simulink model "CAMFC2_04_Quad_03_R2017a"  (R2017a)
settings: Solver=ode45  StartTime=0.0  StopTime=360  RelTol=1e-3  EnableMultiTasking=on
InitFcn:
  | constant_CAMFC2_04_Quad_03
values from neighbouring files (symbols this model uses):
  alpha = 0.1    [constant_CAMFC2_01_WMR01.m]    (also in constant_CAMFC2_04_Comp.m = 0.01; constant_CAMFC2_04_Quad_03.m; constant_CAMFC2_04_Simple.m = 0.01; constant_CAMFC2_04_Simple_DoubleIntegrator.m = 0.01)
  AN = [     0 1 0 0 ... (first row only)    [constant_CAMFC2_01_WMR01.m]    (also in constant_CAMFC2_04_Comp.m = [     0 1 0 0 1; constant_CAMFC2_04_Quad_03.m; constant_CAMFC2_04_Simple.m; constant_CAMFC2_04_Simple_DoubleIntegrator.m)
  B = eye(n)    [constant_CAMFC2_01_WMR01.m]    (also in constant_CAMFC2_04_Quad_03.m; constant_CAMFC2_Quad_New_02.m)
  BBT_inv = ((B'*B)^(-1))*B'    [constant_CAMFC2_04_Quad_03.m]    (also in constant_CAMFC2_Quad_New_02.m)
  Beta = 0.2    [constant_CAMFC2_04_Quad_03.m]    (also in constant_CAMFC2_Quad_New_02.m = 0.1)
  BN = [     1 0 0 0 ... (first row only)    [constant_CAMFC2_01_WMR01.m]    (also in constant_CAMFC2_04_Comp.m = [     0 0 0 0 0; constant_CAMFC2_04_Quad_03.m; constant_CAMFC2_04_Simple.m; constant_CAMFC2_04_Simple_DoubleIntegrator.m)
  Bv = eye(n0)    [constant_CAMFC2_04_Quad_03.m]
  BvBT_inv = ((Bv'*Bv)^(-1))*Bv'    [constant_CAMFC2_04_Quad_03.m]
  chi = [0 0 0 0 ... (first row only)    [constant_CAMFC2_01_WMR01.m]    (also in constant_CAMFC2_04_Comp.m = X_m*ones(n0,1); constant_CAMFC2_04_Quad_03.m = X_m*ones(n0,1); constant_CAMFC2_04_Simple.m = X_m*ones(n0,1); constant_CAMFC2_04_Simple_DoubleIntegrator.m = X_m*ones(n0,1))
  epsilon_struct = struct('data',epsilon_InitVal)    [constant_CAMFC2_01_WMR01.m]    (also in constant_CAMFC2_04_Comp.m; constant_CAMFC2_04_Quad_03.m; constant_CAMFC2_04_Simple.m; constant_CAMFC2_04_Simple_DoubleIntegrator.m)
  gama1 = 1e4*diag([1e-6*ones(2,1);1e0*ones(2,1)])    [constant_CAMFC2_01_WMR01.m]    (also in constant_CAMFC2_04_Comp.m = 1e+3*diag([1e-6;1e-0]); constant_CAMFC2_04_Quad_03.m = 1e+2*diag(1e-0*ones(n0,1)); constant_CAMFC2_04_Simple.m = 1e+2*diag([1e-0;1e-0]); constant_CAMFC2_04_Simple_Formation.m = 1e+2*diag([1e-0;1e-0]))
  gama2 = 1e-2*diag([1e-6*ones(2,1);1e0*ones(2,1)])    [constant_CAMFC2_01_WMR01.m]    (also in constant_CAMFC2_04_Comp.m = 1e+0*diag([1e-6;1e-0]); constant_CAMFC2_04_Quad_03.m = 1e+0*diag(1e-0*ones(n0,1)); constant_CAMFC2_04_Simple.m = 1e+1*diag([1e-0;1e-0]); constant_CAMFC2_04_Simple_Formation.m = 1e+1*diag([1e-0;1e-0]))
  gamma_0 = 1e+0*diag([1e-0*ones(n0,1);1e-0*ones(n0,1)])    [constant_CAMFC2_04_Quad_03.m]    (also in constant_CAMFC2_Quad_New_02.m = 1e-2*diag([1e-6*ones(n0,1);1e-0*ones(n0,1)]))
  gamma_0v = 1e-0*diag(1e-0*ones(n0,1))    [constant_CAMFC2_04_Quad_03.m]
  gamma_1 = 1e+2*diag([1e-0*ones(n0,1);1e-0*ones(n0,1)])    [constant_CAMFC2_04_Quad_03.m]    (also in constant_CAMFC2_Quad_New_02.m = 1e+1*diag([1e-6*ones(n0,1);1e-0*ones(n0,1)]))
  gamma_1v = 1e+2*diag(1e-0*ones(n0,1))    [constant_CAMFC2_04_Quad_03.m]
  ge = 9.81    [constant_CAMFC2_04_Comp.m]    (also in constant_CAMFC2_04_Quad_03.m; constant_CAMFC2_04_Simple.m; constant_CAMFC2_04_Simple_DoubleIntegrator.m; constant_CAMFC2_04_Simple_DoubleIntegrator_02.m)
  H = L + BN    [constant_CAMFC2_01_WMR01.m]    (also in constant_CAMFC2_04_Comp.m; constant_CAMFC2_04_Quad_03.m; constant_CAMFC2_04_Simple.m; constant_CAMFC2_04_Simple_DoubleIntegrator.m)
  Init_Pos_Dif = 0.0    (= 0)    [constant_CAMFC2_04_Quad_03.m]
  J = 0.01    [constant_CAMFC2_01_WMR01.m]    (also in constant_CAMFC2_04_Quad_03.m = 1.0e-3 * diag([1 1 2],0); constant_CAMFC2_Quad_New_02.m = 1.2416e-3 * diag([1 1 2],0))
  k1 = 1    [constant_CAMFC2_01_WMR01.m]    (also in constant_CAMFC2_04_Comp.m; constant_CAMFC2_04_Quad_03.m = 50; constant_CAMFC2_04_Simple.m; constant_CAMFC2_04_Simple_DoubleIntegrator.m)
  k2 = 1    [constant_CAMFC2_01_WMR01.m]    (also in constant_CAMFC2_04_Comp.m; constant_CAMFC2_04_Quad_03.m; constant_CAMFC2_04_Simple.m; constant_CAMFC2_04_Simple_DoubleIntegrator.m)
  Ka = 0.1    [constant_CAMFC2_04_Quad_03.m]    (also in constant_CAMFC2_Quad_New_02.m = 0.01)
  Kd = 0.1    [constant_CAMFC2_04_Quad_03.m]    (also in constant_CAMFC2_Quad_New_02.m = 0.01)
  m = 6    [constant_CAMFC2_04_Quad_03.m]    (also in constant_CAMFC2_Quad_New_02.m)
  M = 1    [constant_CAMFC2_01_WMR01.m]    (also in constant_CAMFC2_04_Quad_03.m = 2; constant_CAMFC2_Quad_New_02.m = 2)
  N = 4    [constant_CAMFC2_01_WMR01.m]    (also in constant_CAMFC2_04_Comp.m = 5; constant_CAMFC2_04_Quad_03.m; constant_CAMFC2_04_Simple.m; constant_CAMFC2_04_Simple_DoubleIntegrator.m)
  n = 4    [constant_CAMFC2_01_WMR01.m]    (also in constant_CAMFC2_04_Comp.m = 2; constant_CAMFC2_04_Quad_03.m = 6; constant_CAMFC2_04_Simple.m = 2; constant_CAMFC2_04_Simple_DoubleIntegrator.m = 2)
  n0 = 2    [constant_CAMFC2_01_WMR01.m]    (also in constant_CAMFC2_04_Comp.m = 1; constant_CAMFC2_04_Quad_03.m = 3; constant_CAMFC2_04_Simple.m; constant_CAMFC2_04_Simple_DoubleIntegrator.m = 1)
  noise_amp = 0.1    [constant_CAMFC2_04_Quad_03.m]
  noise_frq = 1    [constant_CAMFC2_04_Quad_03.m]
  Observer_Gain = 100    [constant_CAMFC2_01_WMR01.m]    (also in constant_CAMFC2_04_Comp.m = 10; constant_CAMFC2_04_Quad_03.m = 1; constant_CAMFC2_04_Simple.m; constant_CAMFC2_04_Simple_DoubleIntegrator.m)
  Observer_Gain1 = 100    [constant_CAMFC2_01_WMR01.m]    (also in constant_CAMFC2_04_Comp.m = 10; constant_CAMFC2_04_Quad_03.m = 1; constant_CAMFC2_04_Simple.m; constant_CAMFC2_04_Simple_DoubleIntegrator.m)
  P_struct = struct('data',P_InitVal)    [constant_CAMFC2_01_WMR01.m]    (also in constant_CAMFC2_04_Comp.m; constant_CAMFC2_04_Quad_03.m; constant_CAMFC2_04_Simple.m; constant_CAMFC2_04_Simple_DoubleIntegrator.m)
  Q = 1e-0*eye(n)    [constant_CAMFC2_01_WMR01.m]    (also in constant_CAMFC2_04_Comp.m = 1.0e+2*eye(n); constant_CAMFC2_04_Quad_03.m = 1e-0*eye(n0); constant_CAMFC2_04_Simple.m = 1.0e+1*eye(n); constant_CAMFC2_04_Simple_Formation.m = 1.0e+1*eye(n))
  QR = 1e-0*eye(n)    [constant_CAMFC2_04_Quad_03.m]    (also in constant_CAMFC2_Quad_New_02.m = 1e+0*eye(n))
  Qv = 1e-0*eye(n0)    [constant_CAMFC2_04_Quad_03.m]
  R = 1e-0*eye(n)    [constant_CAMFC2_01_WMR01.m]    (also in constant_CAMFC2_04_Quad_03.m; constant_CAMFC2_Quad_New_02.m = 1e+0*eye(n))
  r_formX = 1.0    (= 1)    [constant_CAMFC2_04_Quad_03.m]    (also in constant_CAMFC2_Quad_New_02.m)
  r_formY = 1.0    (= 1)    [constant_CAMFC2_04_Quad_03.m]    (also in constant_CAMFC2_Quad_New_02.m)
  r_formZ = 0.5    [constant_CAMFC2_04_Quad_03.m]    (also in constant_CAMFC2_Quad_New_02.m = 1)
  rho1 = 1e-1    (= 0.1)    [constant_CAMFC2_01_WMR01.m]    (also in constant_CAMFC2_04_Comp.m = 1; constant_CAMFC2_04_Quad_03.m = 1; constant_CAMFC2_04_Simple.m = 1; constant_CAMFC2_04_Simple_DoubleIntegrator.m = 1)
  rho2 = 1e-3    (= 0.001)    [constant_CAMFC2_01_WMR01.m]    (also in constant_CAMFC2_04_Comp.m = 1; constant_CAMFC2_04_Quad_03.m = 1; constant_CAMFC2_04_Simple.m = 1; constant_CAMFC2_04_Simple_DoubleIntegrator.m = 10)
  rho_0 = 1e-0    (= 1)    [constant_CAMFC2_04_Quad_03.m]    (also in constant_CAMFC2_Quad_New_02.m = 0.01)
  rho_0v = 1e-0    (= 1)    [constant_CAMFC2_04_Quad_03.m]
  rho_1 = 1e-0    (= 1)    [constant_CAMFC2_04_Quad_03.m]    (also in constant_CAMFC2_Quad_New_02.m = 0.01)
  rho_1v = 1e-0    (= 1)    [constant_CAMFC2_04_Quad_03.m]
  Rv = 1e-0*eye(n0)    [constant_CAMFC2_04_Quad_03.m]
  T_struct = struct('data',T_InitVal)    [constant_CAMFC2_01_WMR01.m]    (also in constant_CAMFC2_04_Comp.m; constant_CAMFC2_04_Quad_03.m; constant_CAMFC2_04_Simple.m; constant_CAMFC2_04_Simple_DoubleIntegrator.m)
  Upsilon_M = Upsilon_m*ones(n,1)    [constant_CAMFC2_01_WMR01.m]    (also in constant_CAMFC2_04_Comp.m; constant_CAMFC2_04_Quad_03.m = Upsilon_m*ones(n0,1); constant_CAMFC2_04_Simple.m; constant_CAMFC2_04_Simple_DoubleIntegrator.m)
(part 3 of 4)

== matlab function CAMFC2_04_Quad_03_R2017a/Agent #2/Decenteralized Cooperaive Controller #2/Cooperative Position Controller #2/Module to compute Consensus Error #2 ==
  data: T_i input; x input; x0 input; ep output; AN parameter; BN parameter; N parameter; n0 parameter; Agent_Num input
function ep = fcn(T_i,x,x0,AN,BN,N,n0,Agent_Num)

Diff_Star_to0 = (T_i((Agent_Num+1),:))';
Diff_Star_to_Other = (eye(n0) * Diff_Star_to0 * ones(1,N))' - T_i(2:N+1,:);
Diff_Star_to_Other = Diff_Star_to_Other';

xp = zeros(n0,N);
for i=1:N
    xp(1:n0,i) = x((i-1)*n0+1:(i*n0));
end

%%
xp_own = zeros(n0,1);
xp_own(1:n0,1) = xp(1:n0,Agent_Num);

xp0 = x0;

xp_other = zeros(n0,N);
ep = zeros(n0,1);
ep(:,1) = ep(:,1) + ( BN(Agent_Num,Agent_Num)*(-(xp_own-xp0)+Diff_Star_to0) );

for i=1:N        
    xp_other(:,i) = xp(:,i);
    ep(:,1) = ep(:,1) + AN(Agent_Num,i)*(-(xp_own-xp_other(:,i))+Diff_Star_to_Other(:,i));
end

end

== matlab function CAMFC2_04_Quad_03_R2017a/Agent #2/Decenteralized Cooperaive Controller #2/Cooperative Position Controller #2/Observer T#2 ==
  data: T_struct parameter; T input; DT_i output; epsilon input; epsilon_struct parameter; H parameter; BN parameter; AN parameter; T_i input; Omega input; Upsilon_M parameter; epsilon_i output; N parameter; n0 parameter; Agent_Num input; Observer_Gain1 parameter; alpha parameter
function [DT_i,epsilon_i] = fcn(T_struct,T,epsilon,epsilon_struct,H,BN,AN,T_i,Omega, Upsilon_M,N,n0,Agent_Num,Observer_Gain1,alpha)

T_struct(1).data = T.t1;
T_struct(2).data = T.t2;
T_struct(3).data = T.t3;
T_struct(4).data = T.t4;

epsilon_struct(1).data = epsilon.eps1;
epsilon_struct(2).data = epsilon.eps2;
epsilon_struct(3).data = epsilon.eps3;
epsilon_struct(4).data = epsilon.eps4;

epsilon_i = + BN(Agent_Num,Agent_Num)*(T_i - Omega);
Sum2 = zeros(N+1,n0);
for i=1:N
    epsilon_i = epsilon_i + ( AN(Agent_Num,i) * (T_i - T_struct(i).data) );  
    Sum2 = Sum2 + ( H(i,Agent_Num) * epsilon_struct(i).data );
end

Sum21 = abs(Sum2) + alpha;
SGN2 = Sum2./Sum21;

DT_i = -Observer_Gain1*epsilon_i - SGN2*diag(Upsilon_M);

end

== matlab function CAMFC2_04_Quad_03_R2017a/Agent #2/Decenteralized Cooperaive Controller #2/Cooperative Position Controller #2/Observer x0_hat#2 ==
  data: x0_hat input; Dx0_hat_i output; x0_tilde input; H parameter; BN parameter; AN parameter; x0_hat_i input; x0 input; chi parameter; x0_tilde_i output; N parameter; Agent_Num input; Observer_Gain parameter; n0 parameter; alpha parameter
function [Dx0_hat_i,x0_tilde_i] = fcn(x0_hat,x0_tilde,H,BN,AN,x0_hat_i,x0,chi,N,Agent_Num,Observer_Gain,n0,alpha)

x0_tilde_i = + BN(Agent_Num,Agent_Num)*(x0_hat_i - x0);

if n0 == 1
    Sum2 = 0;
    for i=1:N
        x0_tilde_i = x0_tilde_i + ( AN(Agent_Num,i) * (x0_hat_i - x0_hat(i)) );  
        Sum2 = Sum2 + ( H(i,Agent_Num) * x0_tilde(i) );
    end    
else
    Sum2 = zeros(n0,1);
    for i=1:N
        x0_tilde_i = x0_tilde_i + ( AN(Agent_Num,i) * (x0_hat_i - x0_hat(((i-1)*n0+1):n0*i)) );  
        Sum2 = Sum2 + ( H(i,Agent_Num) * x0_tilde(((i-1)*n0+1):n0*i) );
    end
end

Sum21 = abs(Sum2) + alpha;
SGN2 = Sum2./Sum21;

Dx0_hat_i = -Observer_Gain*x0_tilde_i - diag(SGN2)*chi;

end

== matlab function CAMFC2_04_Quad_03_R2017a/Agent #2/Decenteralized Cooperaive Controller #2/Rotational AMFC #2/CARE ==
  data: P input; a_hat input; B parameter; R parameter; DP output; QR parameter
function DP = fcn(P,a_hat,B,R,QR)

DP = a_hat*P + P*a_hat' - P*B*R*B'*P + 2*QR;

end

== matlab function CAMFC2_04_Quad_03_R2017a/Agent #2/Decenteralized Cooperaive Controller #2/Rotational AMFC #2/Differentiator/Sliding differentiator ==
  data: u output; u1 input; e input; k1 parameter; alpha parameter
function u = fcn(u1,e,k1,alpha)

b=k1;

ABS = abs(e);
SGN = e ./ (ABS + alpha);
u = u1 - b*((ABS.^0.5).*SGN); 

end

== matlab function CAMFC2_04_Quad_03_R2017a/Agent #2/Decenteralized Cooperaive Controller #2/Rotational AMFC #2/Differentiator/Sliding differentiator1 ==
  data: Du1 output; e input; k2 parameter; alpha parameter
function Du1 = fcn(e,k2,alpha)

a=k2;

ABS = abs(e);
SGN = e ./ (ABS + alpha);
Du1 = - a*SGN;

end

== matlab function CAMFC2_04_Quad_03_R2017a/Agent #2/Decenteralized Cooperaive Controller #2/Rotational AMFC #2/g-Estimator ==
  data: sigma input; g_hat input; P input; rho_1 parameter; gamma_1 parameter; Dg_hat output
function Dg_hat = fcn(sigma,g_hat,P,rho_1,gamma_1)

Dg_hat = - gamma_1 * P * sigma - rho_1 * gamma_1 * g_hat;

end

== matlab function CAMFC2_04_Quad_03_R2017a/Agent #2/Decenteralized Cooperaive Controller #2/Rotational AMFC #2/A-Estimator ==
  data: sigma input; x input; P input; rho_0 parameter; gamma_0 parameter; Da_hat output; a_hat input
function Da_hat = fcn(sigma,x,P,rho_0,gamma_0,a_hat)

DVa_hat = - gamma_0 * P * diag(sigma) * (x - sigma) - rho_0 * gamma_0 * diag(a_hat);

Da_hat = diag(DVa_hat);

end

== matlab function CAMFC2_04_Quad_03_R2017a/Agent #2/Decenteralized Cooperaive Controller #2/Rotational AMFC #2/main ==
  data: sigma input; zeta input; u output; Dy_d input; R parameter; P input; a_hat input; B parameter; g_hat input; x input; QR parameter; BBT_inv parameter; n parameter
function u = fcn(sigma,zeta,Dy_d,R,P,a_hat,B,g_hat,x,QR,BBT_inv,n)

u1 = (1/2) * R * B' * P * sigma;
u2 = BBT_inv * (Dy_d - a_hat*x + (eye(n) + 2*(((P)^(-1)*QR)) + a_hat)*sigma - g_hat - zeta) - (3/4) * R * B' * P * sigma;

u = u1 + u2;

end

== matlab function CAMFC2_04_Quad_03_R2017a/Agent #2/Decenteralized Cooperaive Controller #2/Rotational AMFC #2/variable change ==
  data: X input; Xd input; x_mod output; u input; xd_mod output; e_mod output
function [x_mod,xd_mod,e_mod] = fcn(X,Xd,u)

x_mod = X;

xd_mod = [Xd;u(1:3)];

e_mod = xd_mod - x_mod;


end

== matlab function CAMFC2_04_Quad_03_R2017a/Agent #2/Decenteralized Cooperaive Controller #2/Velocity AMFC #2/A-Estimator  ==
  data: sigma input; x input; P input; rho_0v parameter; gamma_0v parameter; Da_hat output; a_hat input
function Da_hat = fcn(sigma,x,P,rho_0v,gamma_0v,a_hat)

DVa_hat = - gamma_0v * P * diag(sigma) * (x - sigma) - rho_0v * gamma_0v * diag(a_hat);

Da_hat = diag(DVa_hat);

end

== matlab function CAMFC2_04_Quad_03_R2017a/Agent #2/Decenteralized Cooperaive Controller #2/Velocity AMFC #2/CARE ==
  data: P input; a_hat input; Bv parameter; Rv parameter; DP output; Qv parameter
function DP = fcn(P,a_hat,Bv,Rv,Qv)

DP = a_hat*P + P*a_hat' - P*Bv*Rv*Bv'*P + 2*Qv;

end

== matlab function CAMFC2_04_Quad_03_R2017a/Agent #2/Decenteralized Cooperaive Controller #2/Velocity AMFC #2/Differentiator/Sliding differentiator ==
  data: u output; u1 input; e input; k1 parameter; alpha parameter
function u = fcn(u1,e,k1,alpha)

b=k1;

ABS = abs(e);
SGN = e ./ (ABS + alpha);
u = u1 - b*((ABS.^0.5).*SGN); 

end

== matlab function CAMFC2_04_Quad_03_R2017a/Agent #2/Decenteralized Cooperaive Controller #2/Velocity AMFC #2/Differentiator/Sliding differentiator1 ==
  data: Du1 output; e input; k2 parameter; alpha parameter
function Du1 = fcn(e,k2,alpha)

a=k2;

ABS = abs(e);
SGN = e ./ (ABS + alpha);
Du1 = - a*SGN;

end

== matlab function CAMFC2_04_Quad_03_R2017a/Agent #2/Decenteralized Cooperaive Controller #2/Velocity AMFC #2/g-Estimator ==
  data: sigma input; g_hat input; P input; rho_1v parameter; gamma_1v parameter; Dg_hat output
function Dg_hat = fcn(sigma,g_hat,P,rho_1v,gamma_1v)

Dg_hat = - gamma_1v * P * sigma - rho_1v * gamma_1v * g_hat;

end

== matlab function CAMFC2_04_Quad_03_R2017a/Agent #2/Decenteralized Cooperaive Controller #2/Velocity AMFC #2/main ==
  data: sigma input; zeta input; u output; Dy_d input; Rv parameter; P input; a_hat input; Bv parameter; g_hat input; x input; Qv parameter; BvBT_inv parameter; n0 parameter
function u = fcn(sigma,zeta,Dy_d,Rv,P,a_hat,Bv,g_hat,x,Qv,BvBT_inv,n0)

u1 = (1/2) * Rv * Bv' * P * sigma;
u2 = BvBT_inv * (Dy_d - a_hat*x + (eye(n0) + 2*(((P)^(-1)*Qv)) + a_hat)*sigma - g_hat - zeta) - (3/4) * Rv * Bv' * P * sigma;

u = u1 + u2;

end

== matlab function CAMFC2_04_Quad_03_R2017a/Agent #2/Decenteralized Cooperaive Controller #2/Velocity AMFC #2/variable change ==
  data: X input; Xd input; x_mod output; xd_mod output; e_mod output
function [x_mod,xd_mod,e_mod] = fcn(X,Xd)

x_mod = X;
xd_mod = Xd;
e_mod = xd_mod - x_mod;

end

== matlab function CAMFC2_04_Quad_03_R2017a/Agent #2/Plant #2/MATLAB Function ==
  data: XT_V input; XR input; U input; t input; DP output; Dv output; Kd parameter; Ka parameter; M parameter; J parameter; ge parameter; DXR output; noise_amp parameter; noise_frq parameter
function [DP,Dv,DXR] = fcn(XT_V,XR,U,t,Kd,Ka,M,J,ge,noise_amp, noise_frq)

phi = XR(1);
theta = XR(2);
psi = XR(3);

Rq = [cos(psi)*cos(theta) -sin(psi)*cos(phi)+cos(psi)*sin(theta)*sin(phi) sin(psi)*sin(phi)+cos(psi)*sin(theta)*cos(phi);
    sin(psi)*cos(theta) cos(psi)*cos(phi)+sin(psi)*sin(theta)*sin(phi) -cos(psi)*sin(phi)+sin(psi)*sin(theta)*cos(phi);
    -sin(theta) cos(theta)*sin(phi) cos(theta)*cos(phi)]; 

R_omega = [1 0 -sin(theta);
    0 cos(phi) cos(theta)*sin(phi);
    0 -sin(phi) cos(theta)*cos(phi)];

EXT_PRD = External_Product3(XR(4:6),(J*XR(4:6)));

FTT = Rq * [0;0;U(1)];
TTT = U(2:4);

DP = XT_V;
DPHI = (R_omega)^(-1) * XR(4:6); 
Dv = (1/M)*(FTT - Kd*XT_V - M*[0;0;ge] + Rq*(noise_amp*sin(noise_frq*t))*[0;0;1]); 
Dw = (J^(-1))*(TTT - Ka*XR(4:6) - EXT_PRD + (noise_amp*sin(noise_frq*t)*[1;1;1]));
DXR = [DPHI;Dw];

end

== matlab function CAMFC2_04_Quad_03_R2017a/Agent #3/Decenteralized Cooperaive Controller #3/Controller to Motors #3 ==
  data: u output; uT input; uR input
function u = fcn(uT,uR)

y1 = uR(4);
y2 = uR(5);
y3 = uR(6);

Y = [uT;y1;y2;y3];

u = Y;

end

== matlab function CAMFC2_04_Quad_03_R2017a/Agent #3/Decenteralized Cooperaive Controller #3/Cooperative Position Controller #3/Adaptive Law A#3 ==
  data: Agent_Num input; P input; A_hat input; gama2 parameter; rho2 parameter; T_i input; e input; DA_hat output; H parameter; N parameter; x0_hat_i input; P_struct parameter; n0 parameter
function DA_hat = fcn(Agent_Num,P,A_hat,gama2,rho2,T_i,e,H,N,x0_hat_i,P_struct,n0)

%% 
c_i = T_i(1,:)' - T_i(Agent_Num+1,:)' - x0_hat_i;

%%
vA_hat = diag(A_hat);

P_struct(1).data = P.p1;
P_struct(2).data = P.p2;
P_struct(3).data = P.p3;
P_struct(4).data = P.p4;

Sum = zeros(n0,1);
for i=1:N  
    Sum = Sum + (H(Agent_Num,i) * P_struct(i).data * e((i-1)*n0+1:(i*n0),1)); %Adaptive law
end
    
DvA_hat = +gama2*diag(c_i)*Sum - (rho2*gama2*vA_hat);

DA_hat = diag(DvA_hat);

end

== matlab function CAMFC2_04_Quad_03_R2017a/Agent #3/Decenteralized Cooperaive Controller #3/Cooperative Position Controller #3/Adaptive Law g#1 ==
  data: Agent_Num input; g_hat input; gama1 parameter; rho1 parameter; P input; P_struct parameter; Dg_hat output; e input; H parameter; N parameter; n0 parameter
function Dg_hat = fcn(Agent_Num,g_hat,gama1,rho1,P,P_struct,e,H,N,n0)

P_struct(1).data = P.p1;
P_struct(2).data = P.p2;
P_struct(3).data = P.p3;
P_struct(4).data = P.p4;

Sum = zeros(n0,1);
for i=1:N  
    Sum = Sum + (H(Agent_Num,i) * P_struct(i).data * e((i-1)*n0+1:(i*n0),1)); %Adaptive law
end
    
Dg_hat = -gama1*Sum - (rho1*gama1*g_hat);

end

== matlab function CAMFC2_04_Quad_03_R2017a/Agent #3/Decenteralized Cooperaive Controller #3/Cooperative Position Controller #3/DRE3/MATLAB Function ==
  data: inp input; otp output
function otp = fcn(inp)

otp = diag(inp);

end

== matlab function CAMFC2_04_Quad_03_R2017a/Agent #3/Decenteralized Cooperaive Controller #3/Cooperative Position Controller #3/DRE3/MATLAB Function1 ==
  data: inp input; otp output
function otp = fcn(inp)

otp = diag(inp);

end

== matlab function CAMFC2_04_Quad_03_R2017a/Agent #1/Decenteralized Cooperaive Controller #1/Rotational AMFC #1/CARE ==
  data: P input; a_hat input; B parameter; R parameter; DP output; QR parameter
function DP = fcn(P,a_hat,B,R,QR)

DP = a_hat*P + P*a_hat' - P*B*R*B'*P + 2*QR;

end

== matlab function CAMFC2_04_Quad_03_R2017a/Agent #3/Decenteralized Cooperaive Controller #3/Cooperative Position Controller #3/DRE3/P1/DLE1 ==
  data: a_hat input; b output; Agent_Num input; State_Num input; H parameter; Q parameter
function b = fcn(a_hat,Agent_Num,State_Num, H, Q)

h = H(Agent_Num,Agent_Num);
q = Q(State_Num,State_Num);
Delta = (a_hat^2) + (2*q*h);
b = 2*sqrt(Delta);

end

== matlab function CAMFC2_04_Quad_03_R2017a/Data Bus /Translational Log/For matrix Plot1/MATLAB Function ==
  data: u input; y output
function y = fcn(u)
S1 = size(u,1);
S2 = size(u,2);

y = zeros(S1*S2,1);
num = 0;
for i=1:S1
    for j=1:S2
        num = num + 1;
        y(num,1) = u(i,j);
    end
end

end

== matlab function CAMFC2_04_Quad_03_R2017a/Data Bus /Translational Log/For matrix Plot2/MATLAB Function ==
  data: u input; y output
function y = fcn(u)
S1 = size(u,1);
S2 = size(u,2);

y = zeros(S1*S2,1);
num = 0;
for i=1:S1
    for j=1:S2
        num = num + 1;
        y(num,1) = u(i,j);
    end
end

end

== matlab function CAMFC2_04_Quad_03_R2017a/Data Bus /Translational Log/For matrix Plot3/MATLAB Function ==
  data: u input; y output
function y = fcn(u)
S1 = size(u,1);
S2 = size(u,2);

y = zeros(S1*S2,1);
num = 0;
for i=1:S1
    for j=1:S2
        num = num + 1;
        y(num,1) = u(i,j);
    end
end

end

== matlab function CAMFC2_04_Quad_03_R2017a/Data Bus /Translational Log/For matrix Plot4/MATLAB Function ==
  data: u input; y output
function y = fcn(u)
S1 = size(u,1);
S2 = size(u,2);

y = zeros(S1*S2,1);
num = 0;
for i=1:S1
    for j=1:S2
        num = num + 1;
        y(num,1) = u(i,j);
    end
end

end

== matlab function CAMFC2_04_Quad_03_R2017a/Data Bus /Translational Log/For matrix Plot5/MATLAB Function ==
  data: u input; y output
function y = fcn(u)
S1 = size(u,1);
S2 = size(u,2);

y = zeros(S1*S2,1);
num = 0;
for i=1:S1
    for j=1:S2
        num = num + 1;
        y(num,1) = u(i,j);
    end
end

end

== matlab function CAMFC2_04_Quad_03_R2017a/Data Bus /Translational Log/For matrix Plot6/MATLAB Function ==
  data: u input; y output
function y = fcn(u)
S1 = size(u,1);
S2 = size(u,2);

y = zeros(S1*S2,1);
num = 0;
for i=1:S1
    for j=1:S2
        num = num + 1;
        y(num,1) = u(i,j);
    end
end

end

== matlab function CAMFC2_04_Quad_03_R2017a/Data Bus /Translational Log/For matrix Plot7/MATLAB Function ==
  data: u input; y output
function y = fcn(u)
S1 = size(u,1);
S2 = size(u,2);

y = zeros(S1*S2,1);
num = 0;
for i=1:S1
    for j=1:S2
        num = num + 1;
        y(num,1) = u(i,j);
    end
end

end

== matlab function CAMFC2_04_Quad_03_R2017a/Data Bus /Observers Log/For matrix Plot8/MATLAB Function ==
  data: u input; y output
function y = fcn(u)
S1 = size(u,1);
S2 = size(u,2);

y = zeros(S1*S2,1);
num = 0;
for i=1:S1
    for j=1:S2
        num = num + 1;
        y(num,1) = u(i,j);
    end
end

end

== matlab function CAMFC2_04_Quad_03_R2017a/Data Bus /Observers Log/For matrix Plot9/MATLAB Function ==
  data: u input; y output
function y = fcn(u)
S1 = size(u,1);
S2 = size(u,2);

y = zeros(S1*S2,1);
num = 0;
for i=1:S1
    for j=1:S2
        num = num + 1;
        y(num,1) = u(i,j);
    end
end

end

== matlab function CAMFC2_04_Quad_03_R2017a/Agent #3/Decenteralized Cooperaive Controller #3/Cooperative Position Controller #3/DRE3/P1/DRE2 ==
  data: Agent_Num input; State_Num input; a_hat input; p output; val_exp input; H parameter; Q parameter
function p = fcn(Agent_Num,State_Num,a_hat,val_exp,H, Q)

p_init = 1;
h = H(Agent_Num,Agent_Num);
q = Q(State_Num,State_Num);
Delta = (a_hat^2) + (2*q*h);
p0 = (1/h) * (a_hat - sqrt(Delta));
w0 = 1 / (p_init - p0);
b = 2*sqrt(Delta);
w = (h/b) + (w0 - (h/b))*exp(val_exp);
p = p0 + (1/w);

end

== matlab function CAMFC2_04_Quad_03_R2017a/Agent #3/Decenteralized Cooperaive Controller #3/Cooperative Position Controller #3/DRE3/P2/DLE1 ==
  data: a_hat input; b output; Agent_Num input; State_Num input; H parameter; Q parameter
function b = fcn(a_hat,Agent_Num,State_Num, H, Q)

h = H(Agent_Num,Agent_Num);
q = Q(State_Num,State_Num);
Delta = (a_hat^2) + (2*q*h);
b = 2*sqrt(Delta);

end

== matlab function CAMFC2_04_Quad_03_R2017a/Data Bus /Translational Log/For matrix Plot/MATLAB Function ==
  data: u input; y output
function y = fcn(u)
S1 = size(u,1);
S2 = size(u,2);

y = zeros(S1*S2,1);
num = 0;
for i=1:S1
    for j=1:S2
        num = num + 1;
        y(num,1) = u(i,j);
    end
end

end

== matlab function CAMFC2_04_Quad_03_R2017a/Data Bus /Observers Log/For matrix Plot10/MATLAB Function ==
  data: u input; y output
function y = fcn(u)
S1 = size(u,1);
S2 = size(u,2);

y = zeros(S1*S2,1);
num = 0;
for i=1:S1
    for j=1:S2
        num = num + 1;
        y(num,1) = u(i,j);
    end
end

end

== matlab function CAMFC2_04_Quad_03_R2017a/Data Bus /Observers Log/For matrix Plot11/MATLAB Function ==
  data: u input; y output
function y = fcn(u)
S1 = size(u,1);
S2 = size(u,2);

y = zeros(S1*S2,1);
num = 0;
for i=1:S1
    for j=1:S2
        num = num + 1;
        y(num,1) = u(i,j);
    end
end

end

== matlab function CAMFC2_04_Quad_03_R2017a/Data Bus /Observers Log/For matrix Plot12/MATLAB Function ==
  data: u input; y output
function y = fcn(u)
S1 = size(u,1);
S2 = size(u,2);

y = zeros(S1*S2,1);
num = 0;
for i=1:S1
    for j=1:S2
        num = num + 1;
        y(num,1) = u(i,j);
    end
end

end

== matlab function CAMFC2_04_Quad_03_R2017a/Agent #3/Decenteralized Cooperaive Controller #3/Cooperative Position Controller #3/DRE3/P2/DRE2 ==
  data: Agent_Num input; State_Num input; a_hat input; p output; val_exp input; H parameter; Q parameter
function p = fcn(Agent_Num,State_Num,a_hat,val_exp,H, Q)

p_init = 1;
h = H(Agent_Num,Agent_Num);
q = Q(State_Num,State_Num);
Delta = (a_hat^2) + (2*q*h);
p0 = (1/h) * (a_hat - sqrt(Delta));
w0 = 1 / (p_init - p0);
b = 2*sqrt(Delta);
w = (h/b) + (w0 - (h/b))*exp(val_exp);
p = p0 + (1/w);

end

== matlab function CAMFC2_04_Quad_03_R2017a/Data Bus /Observers Log/For matrix Plot13/MATLAB Function ==
  data: u input; y output
function y = fcn(u)
S1 = size(u,1);
S2 = size(u,2);

y = zeros(S1*S2,1);
num = 0;
for i=1:S1
    for j=1:S2
        num = num + 1;
        y(num,1) = u(i,j);
    end
end

end

== matlab function CAMFC2_04_Quad_03_R2017a/Agent #3/Decenteralized Cooperaive Controller #3/Cooperative Position Controller #3/DRE3/P3/DLE1 ==
  data: a_hat input; b output; Agent_Num input; State_Num input; H parameter; Q parameter
function b = fcn(a_hat,Agent_Num,State_Num, H, Q)

h = H(Agent_Num,Agent_Num);
q = Q(State_Num,State_Num);
Delta = (a_hat^2) + (2*q*h);
b = 2*sqrt(Delta);

end

== matlab function CAMFC2_04_Quad_03_R2017a/Agent #1/Decenteralized Cooperaive Controller #1/Cooperative Position Controller #1/DRE1/P2/DLE1 ==
  data: a_hat input; b output; Agent_Num input; State_Num input; H parameter; Q parameter
function b = fcn(a_hat,Agent_Num,State_Num, H, Q)

h = H(Agent_Num,Agent_Num);
q = Q(State_Num,State_Num);
Delta = (a_hat^2) + (2*q*h);
b = 2*sqrt(Delta);

end

== matlab function CAMFC2_04_Quad_03_R2017a/Data Bus /Observers Log/For matrix Plot14/MATLAB Function ==
  data: u input; y output
function y = fcn(u)
S1 = size(u,1);
S2 = size(u,2);

y = zeros(S1*S2,1);
num = 0;
for i=1:S1
    for j=1:S2
        num = num + 1;
        y(num,1) = u(i,j);
    end
end

end

== matlab function CAMFC2_04_Quad_03_R2017a/Data Bus /Observers Log/For matrix Plot15/MATLAB Function ==
  data: u input; y output
function y = fcn(u)
S1 = size(u,1);
S2 = size(u,2);

y = zeros(S1*S2,1);
num = 0;
for i=1:S1
    for j=1:S2
        num = num + 1;
        y(num,1) = u(i,j);
    end
end

end

== matlab function CAMFC2_04_Quad_03_R2017a/Agent #1/Decenteralized Cooperaive Controller #1/Cooperative Position Controller #1/DRE1/P2/DRE2 ==
  data: Agent_Num input; State_Num input; a_hat input; p output; val_exp input; H parameter; Q parameter
function p = fcn(Agent_Num,State_Num,a_hat,val_exp,H, Q)

p_init = 1;
h = H(Agent_Num,Agent_Num);
q = Q(State_Num,State_Num);
Delta = (a_hat^2) + (2*q*h);
p0 = (1/h) * (a_hat - sqrt(Delta));
w0 = 1 / (p_init - p0);
b = 2*sqrt(Delta);
w = (h/b) + (w0 - (h/b))*exp(val_exp);
p = p0 + (1/w);

end

== matlab function CAMFC2_04_Quad_03_R2017a/Data Bus /Reference Trajectory/MATLAB Function ==
  data: r_formZ_inp input; Omega output; r_formX_inp input; r_formY_inp input
function Omega = fcn(r_formZ_inp, r_formX_inp, r_formY_inp)

Delta_form = [...
    +r_formX_inp +r_formY_inp +r_formZ_inp;
    -r_formX_inp +r_formY_inp +2*r_formZ_inp;
    -r_formX_inp -r_formY_inp +3*r_formZ_inp;
    +r_formX_inp -r_formY_inp +4*r_formZ_inp];

Omega = [0 0 0;
    Delta_form];

end

== matlab function CAMFC2_04_Quad_03_R2017a/Agent #1/Decenteralized Cooperaive Controller #1/Rotational AMFC #1/Differentiator/Sliding differentiator ==
  data: u output; u1 input; e input; k1 parameter; alpha parameter
function u = fcn(u1,e,k1,alpha)

b=k1;

ABS = abs(e);
SGN = e ./ (ABS + alpha);
u = u1 - b*((ABS.^0.5).*SGN); 

end

== matlab function CAMFC2_04_Quad_03_R2017a/Agent #3/Decenteralized Cooperaive Controller #3/Cooperative Position Controller #3/DRE3/P3/DRE2 ==
  data: Agent_Num input; State_Num input; a_hat input; p output; val_exp input; H parameter; Q parameter
function p = fcn(Agent_Num,State_Num,a_hat,val_exp,H, Q)

p_init = 1;
h = H(Agent_Num,Agent_Num);
q = Q(State_Num,State_Num);
Delta = (a_hat^2) + (2*q*h);
p0 = (1/h) * (a_hat - sqrt(Delta));
w0 = 1 / (p_init - p0);
b = 2*sqrt(Delta);
w = (h/b) + (w0 - (h/b))*exp(val_exp);
p = p0 + (1/w);

end

== matlab function CAMFC2_04_Quad_03_R2017a/Agent #3/Decenteralized Cooperaive Controller #3/Cooperative Position Controller #3/Differentiator2/Sliding differentiator ==
  data: u output; u1 input; e input; k1 parameter; alpha parameter
function u = fcn(u1,e,k1,alpha)

b=k1;

ABS = abs(e);
SGN = e ./ (ABS + alpha);
u = u1 - b*((ABS.^0.5).*SGN); 

end

== matlab function CAMFC2_04_Quad_03_R2017a/Agent #3/Decenteralized Cooperaive Controller #3/Cooperative Position Controller #3/Differentiator2/Sliding differentiator1 ==
  data: Du1 output; e input; k2 parameter; alpha parameter
function Du1 = fcn(e,k2,alpha)

a=k2;

ABS = abs(e);
SGN = e ./ (ABS + alpha);
Du1 = - a*SGN;

end

== matlab function CAMFC2_04_Quad_03_R2017a/Agent #3/Decenteralized Cooperaive Controller #3/Cooperative Position Controller #3/Main Controller #3 ==
  data: A_hat_i input; DT_i input; T_i input; g_hat_i input; Agent_Num input; U output; x0_hat_i input; Dx0_hat_i input; P_i input; e_i input
function U = fcn(A_hat_i,DT_i,T_i,g_hat_i,Agent_Num,x0_hat_i,Dx0_hat_i,P_i,e_i)

%%
c_i = T_i(1,:)' - T_i(Agent_Num+1,:)' - x0_hat_i;
Dc_i = DT_i(1,:)' - DT_i(Agent_Num+1,:)' - Dx0_hat_i;

%%
U1 = A_hat_i * c_i; %linear terms compensation
U2 = - g_hat_i; %nonlinear terms compensation 
U3 = - Dc_i; %Derivative of Formation parameters and the virtual leader's states 
U4 = + 0.5 * P_i * e_i;

U = U1 + U2 + U3 + U4;

end

== matlab function CAMFC2_04_Quad_03_R2017a/Agent #1/Decenteralized Cooperaive Controller #1/Controller Interpreter #1 ==
  data: ut_i input; uT_i output; PHI_d_i output; thresh_euler parameter
function [uT_i,PHI_d_i] = fcn(ut_i,thresh_euler)

%%
f0 = sqrt((ut_i(1)^2)+(ut_i(2)^2)+(ut_i(3)^2));
psi_d = 0;
phi_d = asin( min(max(((sin(psi_d)*ut_i(1) - cos(psi_d)*ut_i(2)) / (f0+1e-3)),-1),1) );
theta_d = atan2( (cos(psi_d)*ut_i(1) + sin(psi_d)*ut_i(2)) , (ut_i(3)+1e-3) );
if (abs(theta_d)<thresh_euler)
    theta_d = 0;
end
if (abs(phi_d)<thresh_euler)
    phi_d = 0;
end
PHI_d_i = [phi_d;theta_d;psi_d]; 
uT_i = f0;

end

== matlab function CAMFC2_04_Quad_03_R2017a/Agent #1/Decenteralized Cooperaive Controller #1/Rotational AMFC #1/Differentiator/Sliding differentiator1 ==
  data: Du1 output; e input; k2 parameter; alpha parameter
function Du1 = fcn(e,k2,alpha)

a=k2;

ABS = abs(e);
SGN = e ./ (ABS + alpha);
Du1 = - a*SGN;

end

== matlab function CAMFC2_04_Quad_03_R2017a/Agent #1/Decenteralized Cooperaive Controller #1/Rotational AMFC #1/g-Estimator ==
  data: sigma input; g_hat input; P input; rho_1 parameter; gamma_1 parameter; Dg_hat output
function Dg_hat = fcn(sigma,g_hat,P,rho_1,gamma_1)

Dg_hat = - gamma_1 * P * sigma - rho_1 * gamma_1 * g_hat;

end

== matlab function CAMFC2_04_Quad_03_R2017a/Agent #1/Decenteralized Cooperaive Controller #1/Rotational AMFC #1/g-Estimator1 ==
  data: sigma input; x input; P input; rho_0 parameter; gamma_0 parameter; Da_hat output; a_hat input
function Da_hat = fcn(sigma,x,P,rho_0,gamma_0,a_hat)

DVa_hat = - gamma_0 * P * diag(sigma) * (x - sigma) - rho_0 * gamma_0 * diag(a_hat);

Da_hat = diag(DVa_hat);

end

== matlab function CAMFC2_04_Quad_03_R2017a/Agent #1/Decenteralized Cooperaive Controller #1/Rotational AMFC #1/main ==
  data: sigma input; zeta input; u output; Dy_d input; R parameter; P input; a_hat input; B parameter; g_hat input; x input; QR parameter; BBT_inv parameter; n parameter
function u = fcn(sigma,zeta,Dy_d,R,P,a_hat,B,g_hat,x,QR,BBT_inv,n)

u1 = (1/2) * R * B' * P * sigma;
u2 = BBT_inv * (Dy_d - a_hat*x + (eye(n) + 2*(((P)^(-1)*QR)) + a_hat)*sigma - g_hat - zeta) - (3/4) * R * B' * P * sigma;

u = u1 + u2;

end

== matlab function CAMFC2_04_Quad_03_R2017a/Agent #1/Decenteralized Cooperaive Controller #1/Rotational AMFC #1/variable change ==
  data: X input; Xd input; x_mod output; u input; xd_mod output; e_mod output
function [x_mod,xd_mod,e_mod] = fcn(X,Xd,u)

x_mod = X;

xd_mod = [Xd;u(1:3)];

e_mod = xd_mod - x_mod;


end

== matlab function CAMFC2_04_Quad_03_R2017a/Agent #3/Decenteralized Cooperaive Controller #3/Cooperative Position Controller #3/Module to compute Consensus Error #3 ==
  data: T_i input; x input; x0 input; ep output; AN parameter; BN parameter; N parameter; n0 parameter; Agent_Num input
function ep = fcn(T_i,x,x0,AN,BN,N,n0,Agent_Num)

Diff_Star_to0 = (T_i((Agent_Num+1),:))';
Diff_Star_to_Other = (eye(n0) * Diff_Star_to0 * ones(1,N))' - T_i(2:N+1,:);
Diff_Star_to_Other = Diff_Star_to_Other';

xp = zeros(n0,N);
for i=1:N
    xp(1:n0,i) = x((i-1)*n0+1:(i*n0));
end

%%
xp_own = zeros(n0,1);
xp_own(1:n0,1) = xp(1:n0,Agent_Num);

xp0 = x0;

xp_other = zeros(n0,N);
ep = zeros(n0,1);
ep(:,1) = ep(:,1) + ( BN(Agent_Num,Agent_Num)*(-(xp_own-xp0)+Diff_Star_to0) );

for i=1:N        
    xp_other(:,i) = xp(:,i);
    ep(:,1) = ep(:,1) + AN(Agent_Num,i)*(-(xp_own-xp_other(:,i))+Diff_Star_to_Other(:,i));
end

end

== matlab function CAMFC2_04_Quad_03_R2017a/Agent #3/Decenteralized Cooperaive Controller #3/Cooperative Position Controller #3/Observer T#3 ==
  data: T_struct parameter; T input; DT_i output; epsilon input; epsilon_struct parameter; H parameter; BN parameter; AN parameter; T_i input; Omega input; Upsilon_M parameter; epsilon_i output; N parameter; n0 parameter; Agent_Num input; Observer_Gain1 parameter; alpha parameter
function [DT_i,epsilon_i] = fcn(T_struct,T,epsilon,epsilon_struct,H,BN,AN,T_i,Omega, Upsilon_M,N,n0,Agent_Num,Observer_Gain1,alpha)

T_struct(1).data = T.t1;
T_struct(2).data = T.t2;
T_struct(3).data = T.t3;
T_struct(4).data = T.t4;

epsilon_struct(1).data = epsilon.eps1;
epsilon_struct(2).data = epsilon.eps2;
epsilon_struct(3).data = epsilon.eps3;
epsilon_struct(4).data = epsilon.eps4;

epsilon_i = + BN(Agent_Num,Agent_Num)*(T_i - Omega);
Sum2 = zeros(N+1,n0);
for i=1:N
    epsilon_i = epsilon_i + ( AN(Agent_Num,i) * (T_i - T_struct(i).data) );  
    Sum2 = Sum2 + ( H(i,Agent_Num) * epsilon_struct(i).data );
end

Sum21 = abs(Sum2) + alpha;
SGN2 = Sum2./Sum21;

DT_i = -Observer_Gain1*epsilon_i - SGN2*diag(Upsilon_M);

end

== matlab function CAMFC2_04_Quad_03_R2017a/Agent #3/Decenteralized Cooperaive Controller #3/Cooperative Position Controller #3/Observer x0_hat#3 ==
  data: x0_hat input; Dx0_hat_i output; x0_tilde input; H parameter; BN parameter; AN parameter; x0_hat_i input; x0 input; chi parameter; x0_tilde_i output; N parameter; Agent_Num input; Observer_Gain parameter; n0 parameter; alpha parameter
function [Dx0_hat_i,x0_tilde_i] = fcn(x0_hat,x0_tilde,H,BN,AN,x0_hat_i,x0,chi,N,Agent_Num,Observer_Gain,n0,alpha)

x0_tilde_i = + BN(Agent_Num,Agent_Num)*(x0_hat_i - x0);

if n0 == 1
    Sum2 = 0;
    for i=1:N
        x0_tilde_i = x0_tilde_i + ( AN(Agent_Num,i) * (x0_hat_i - x0_hat(i)) );  
        Sum2 = Sum2 + ( H(i,Agent_Num) * x0_tilde(i) );
    end    
else
    Sum2 = zeros(n0,1);
    for i=1:N
        x0_tilde_i = x0_tilde_i + ( AN(Agent_Num,i) * (x0_hat_i - x0_hat(((i-1)*n0+1):n0*i)) );  
        Sum2 = Sum2 + ( H(i,Agent_Num) * x0_tilde(((i-1)*n0+1):n0*i) );
    end
end

Sum21 = abs(Sum2) + alpha;
SGN2 = Sum2./Sum21;

Dx0_hat_i = -Observer_Gain*x0_tilde_i - diag(SGN2)*chi;

end

== matlab function CAMFC2_04_Quad_03_R2017a/Agent #3/Decenteralized Cooperaive Controller #3/Rotational AMFC #3/CARE ==
  data: P input; a_hat input; B parameter; R parameter; DP output; QR parameter
function DP = fcn(P,a_hat,B,R,QR)

DP = a_hat*P + P*a_hat' - P*B*R*B'*P + 2*QR;

end

== matlab function CAMFC2_04_Quad_03_R2017a/Data Bus /Rotational Log/For matrix Plot/MATLAB Function ==
  data: u input; y output
function y = fcn(u)
S1 = size(u,1);
S2 = size(u,2);

y = zeros(S1*S2,1);
num = 0;
for i=1:S1
    for j=1:S2
        num = num + 1;
        y(num,1) = u(i,j);
    end
end

end

== matlab function CAMFC2_04_Quad_03_R2017a/Data Bus /Rotational Log/For matrix Plot1/MATLAB Function ==
  data: u input; y output
function y = fcn(u)
S1 = size(u,1);
S2 = size(u,2);

y = zeros(S1*S2,1);
num = 0;
for i=1:S1
    for j=1:S2
        num = num + 1;
        y(num,1) = u(i,j);
    end
end

end

== matlab function CAMFC2_04_Quad_03_R2017a/Data Bus /Rotational Log/For matrix Plot2/MATLAB Function ==
  data: u input; y output
function y = fcn(u)
S1 = size(u,1);
S2 = size(u,2);

y = zeros(S1*S2,1);
num = 0;
for i=1:S1
    for j=1:S2
        num = num + 1;
        y(num,1) = u(i,j);
    end
end

end

== matlab function CAMFC2_04_Quad_03_R2017a/Data Bus /Rotational Log/For matrix Plot3/MATLAB Function ==
  data: u input; y output
function y = fcn(u)
S1 = size(u,1);
S2 = size(u,2);

y = zeros(S1*S2,1);
num = 0;
for i=1:S1
    for j=1:S2
        num = num + 1;
        y(num,1) = u(i,j);
    end
end

end

== matlab function CAMFC2_04_Quad_03_R2017a/Data Bus /Rotational Log/For matrix Plot4/MATLAB Function ==
  data: u input; y output
function y = fcn(u)
S1 = size(u,1);
S2 = size(u,2);

y = zeros(S1*S2,1);
num = 0;
for i=1:S1
    for j=1:S2
        num = num + 1;
        y(num,1) = u(i,j);
    end
end

end

== matlab function CAMFC2_04_Quad_03_R2017a/Data Bus /Rotational Log/For matrix Plot5/MATLAB Function ==
  data: u input; y output
function y = fcn(u)
S1 = size(u,1);
S2 = size(u,2);

y = zeros(S1*S2,1);
num = 0;
for i=1:S1
    for j=1:S2
        num = num + 1;
        y(num,1) = u(i,j);
    end
end

end

== matlab function CAMFC2_04_Quad_03_R2017a/Agent #3/Decenteralized Cooperaive Controller #3/Rotational AMFC #3/Differentiator/Sliding differentiator ==
  data: u output; u1 input; e input; k1 parameter; alpha parameter
function u = fcn(u1,e,k1,alpha)

b=k1;

ABS = abs(e);
SGN = e ./ (ABS + alpha);
u = u1 - b*((ABS.^0.5).*SGN); 

end

== matlab function CAMFC2_04_Quad_03_R2017a/Agent #3/Decenteralized Cooperaive Controller #3/Rotational AMFC #3/Differentiator/Sliding differentiator1 ==
  data: Du1 output; e input; k2 parameter; alpha parameter
function Du1 = fcn(e,k2,alpha)

a=k2;

ABS = abs(e);
SGN = e ./ (ABS + alpha);
Du1 = - a*SGN;

end

== matlab function CAMFC2_04_Quad_03_R2017a/Agent #3/Decenteralized Cooperaive Controller #3/Rotational AMFC #3/g-Estimator ==
  data: sigma input; g_hat input; P input; rho_1 parameter; gamma_1 parameter; Dg_hat output
function Dg_hat = fcn(sigma,g_hat,P,rho_1,gamma_1)

Dg_hat = - gamma_1 * P * sigma - rho_1 * gamma_1 * g_hat;

end

== matlab function CAMFC2_04_Quad_03_R2017a/Agent #3/Decenteralized Cooperaive Controller #3/Rotational AMFC #3/A-Estimator ==
  data: sigma input; x input; P input; rho_0 parameter; gamma_0 parameter; Da_hat output; a_hat input
function Da_hat = fcn(sigma,x,P,rho_0,gamma_0,a_hat)

DVa_hat = - gamma_0 * P * diag(sigma) * (x - sigma) - rho_0 * gamma_0 * diag(a_hat);

Da_hat = diag(DVa_hat);

end

== matlab function CAMFC2_04_Quad_03_R2017a/Agent #3/Decenteralized Cooperaive Controller #3/Rotational AMFC #3/main ==
  data: sigma input; zeta input; u output; Dy_d input; R parameter; P input; a_hat input; B parameter; g_hat input; x input; QR parameter; BBT_inv parameter; n parameter
function u = fcn(sigma,zeta,Dy_d,R,P,a_hat,B,g_hat,x,QR,BBT_inv,n)

u1 = (1/2) * R * B' * P * sigma;
u2 = BBT_inv * (Dy_d - a_hat*x + (eye(n) + 2*(((P)^(-1)*QR)) + a_hat)*sigma - g_hat - zeta) - (3/4) * R * B' * P * sigma;

u = u1 + u2;

end

== matlab function CAMFC2_04_Quad_03_R2017a/Data Bus /Rotational Log/For matrix Plot6/MATLAB Function ==
  data: u input; y output
function y = fcn(u)
S1 = size(u,1);
S2 = size(u,2);

y = zeros(S1*S2,1);
num = 0;
for i=1:S1
    for j=1:S2
        num = num + 1;
        y(num,1) = u(i,j);
    end
end

end

== matlab function CAMFC2_04_Quad_03_R2017a/Agent #3/Decenteralized Cooperaive Controller #3/Rotational AMFC #3/variable change ==
  data: X input; Xd input; x_mod output; u input; xd_mod output; e_mod output
function [x_mod,xd_mod,e_mod] = fcn(X,Xd,u)

x_mod = X;

xd_mod = [Xd;u(1:3)];

e_mod = xd_mod - x_mod;


end

== matlab function CAMFC2_04_Quad_03_R2017a/Data Bus /Rotational Log/For matrix Plot7/MATLAB Function ==
  data: u input; y output
function y = fcn(u)
S1 = size(u,1);
S2 = size(u,2);

y = zeros(S1*S2,1);
num = 0;
for i=1:S1
    for j=1:S2
        num = num + 1;
        y(num,1) = u(i,j);
    end
end

end

== matlab function CAMFC2_04_Quad_03_R2017a/Agent #1/Decenteralized Cooperaive Controller #1/Cooperative Position Controller #1/Differentiator2/Sliding differentiator ==
  data: u output; u1 input; e input; k1 parameter; alpha parameter
function u = fcn(u1,e,k1,alpha)

b=k1;

ABS = abs(e);
SGN = e ./ (ABS + alpha);
u = u1 - b*((ABS.^0.5).*SGN); 

end

== matlab function CAMFC2_04_Quad_03_R2017a/Agent #1/Decenteralized Cooperaive Controller #1/Cooperative Position Controller #1/Differentiator2/Sliding differentiator1 ==
  data: Du1 output; e input; k2 parameter; alpha parameter
function Du1 = fcn(e,k2,alpha)

a=k2;

ABS = abs(e);
SGN = e ./ (ABS + alpha);
Du1 = - a*SGN;

end

== matlab function CAMFC2_04_Quad_03_R2017a/Agent #1/Decenteralized Cooperaive Controller #1/Cooperative Position Controller #1/Main Controller #1 ==
  data: A_hat_i input; DT_i input; T_i input; g_hat_i input; Agent_Num input; U output; x0_hat_i input; Dx0_hat_i input; P_i input; e_i input
function U = fcn(A_hat_i,DT_i,T_i,g_hat_i,Agent_Num,x0_hat_i,Dx0_hat_i,P_i,e_i)

%%
c_i = T_i(1,:)' - T_i(Agent_Num+1,:)' - x0_hat_i;
Dc_i = DT_i(1,:)' - DT_i(Agent_Num+1,:)' - Dx0_hat_i;

%%
U1 = A_hat_i * c_i; %linear terms compensation
U2 = - g_hat_i; %nonlinear terms compensation 
U3 = - Dc_i; %Derivative of Formation parameters and the virtual leader's states 
U4 = + 0.5 * P_i * e_i;

U = zeros(3,1) + U1 + U2 + U3 + U4;

end

== matlab function CAMFC2_04_Quad_03_R2017a/Agent #1/Decenteralized Cooperaive Controller #1/Cooperative Position Controller #1/Module to compute Consensus Error #1 ==
  data: T_i input; x input; x0 input; ep output; AN parameter; BN parameter; N parameter; n0 parameter; Agent_Num input
function ep = fcn(T_i,x,x0,AN,BN,N,n0,Agent_Num)

Diff_Star_to0 = (T_i((Agent_Num+1),:))';
Diff_Star_to_Other = (eye(n0) * Diff_Star_to0 * ones(1,N))' - T_i(2:N+1,:);
Diff_Star_to_Other = Diff_Star_to_Other';

xp = zeros(n0,N);
for i=1:N
    xp(1:n0,i) = x((i-1)*n0+1:(i*n0));
end

%%
xp_own = zeros(n0,1);
xp_own(1:n0,1) = xp(1:n0,Agent_Num);

xp0 = x0;

xp_other = zeros(n0,N);
ep = zeros(n0,1);
ep(:,1) = ep(:,1) + ( BN(Agent_Num,Agent_Num)*(-(xp_own-xp0)+Diff_Star_to0) );

for i=1:N        
    xp_other(:,i) = xp(:,i);
    ep(:,1) = ep(:,1) + AN(Agent_Num,i)*(-(xp_own-xp_other(:,i))+Diff_Star_to_Other(:,i));
end

end

== matlab function CAMFC2_04_Quad_03_R2017a/Agent #1/Decenteralized Cooperaive Controller #1/Cooperative Position Controller #1/Observer T#1 ==
  data: T_struct parameter; T input; DT_i output; epsilon input; epsilon_struct parameter; H parameter; BN parameter; AN parameter; T_i input; Omega input; Upsilon_M parameter; epsilon_i output; N parameter; n0 parameter; Agent_Num input; Observer_Gain1 parameter; alpha parameter
function [DT_i,epsilon_i] = fcn(T_struct,T,epsilon,epsilon_struct,H,BN,AN,T_i,Omega, Upsilon_M,N,n0,Agent_Num,Observer_Gain1,alpha)

T_struct(1).data = T.t1;
T_struct(2).data = T.t2;
T_struct(3).data = T.t3;
T_struct(4).data = T.t4;

epsilon_struct(1).data = epsilon.eps1;
epsilon_struct(2).data = epsilon.eps2;
epsilon_struct(3).data = epsilon.eps3;
epsilon_struct(4).data = epsilon.eps4;

epsilon_i = + BN(Agent_Num,Agent_Num)*(T_i - Omega);
Sum2 = zeros(N+1,n0);
for i=1:N
    epsilon_i = epsilon_i + ( AN(Agent_Num,i) * (T_i - T_struct(i).data) );  
    Sum2 = Sum2 + ( H(i,Agent_Num) * epsilon_struct(i).data );
end

Sum21 = abs(Sum2) + alpha;
SGN2 = Sum2./Sum21;

DT_i = -Observer_Gain1*epsilon_i - SGN2*diag(Upsilon_M);

end

== matlab function CAMFC2_04_Quad_03_R2017a/Agent #1/Decenteralized Cooperaive Controller #1/Cooperative Position Controller #1/Observer x0_hat#1 ==
  data: x0_hat input; Dx0_hat_i output; x0_tilde input; H parameter; BN parameter; AN parameter; x0_hat_i input; x0 input; chi parameter; x0_tilde_i output; N parameter; Agent_Num input; Observer_Gain parameter; n0 parameter; alpha parameter
function [Dx0_hat_i,x0_tilde_i] = fcn(x0_hat,x0_tilde,H,BN,AN,x0_hat_i,x0,chi,N,Agent_Num,Observer_Gain,n0,alpha)

x0_tilde_i = + BN(Agent_Num,Agent_Num)*(x0_hat_i - x0);

if n0 == 1
    Sum2 = 0;
    for i=1:N
        x0_tilde_i = x0_tilde_i + ( AN(Agent_Num,i) * (x0_hat_i - x0_hat(i)) );  
        Sum2 = Sum2 + ( H(i,Agent_Num) * x0_tilde(i) );
    end    
else
    Sum2 = zeros(n0,1);
    for i=1:N
        x0_tilde_i = x0_tilde_i + ( AN(Agent_Num,i) * (x0_hat_i - x0_hat(((i-1)*n0+1):n0*i)) );  
        Sum2 = Sum2 + ( H(i,Agent_Num) * x0_tilde(((i-1)*n0+1):n0*i) );
    end
end

Sum21 = abs(Sum2) + alpha;
SGN2 = Sum2./Sum21;

Dx0_hat_i = -Observer_Gain*x0_tilde_i - diag(SGN2)*chi;

end

== matlab function CAMFC2_04_Quad_03_R2017a/Agent #3/Decenteralized Cooperaive Controller #3/Velocity AMFC #3/A-Estimator  ==
  data: sigma input; x input; P input; rho_0v parameter; gamma_0v parameter; Da_hat output; a_hat input
function Da_hat = fcn(sigma,x,P,rho_0v,gamma_0v,a_hat)

DVa_hat = - gamma_0v * P * diag(sigma) * (x - sigma) - rho_0v * gamma_0v * diag(a_hat);

Da_hat = diag(DVa_hat);

end

== matlab function CAMFC2_04_Quad_03_R2017a/Agent #3/Decenteralized Cooperaive Controller #3/Velocity AMFC #3/CARE ==
  data: P input; a_hat input; Bv parameter; Rv parameter; DP output; Qv parameter
function DP = fcn(P,a_hat,Bv,Rv,Qv)

DP = a_hat*P + P*a_hat' - P*Bv*Rv*Bv'*P + 2*Qv;

end

== matlab function CAMFC2_04_Quad_03_R2017a/Agent #3/Decenteralized Cooperaive Controller #3/Velocity AMFC #3/Differentiator/Sliding differentiator ==
  data: u output; u1 input; e input; k1 parameter; alpha parameter
function u = fcn(u1,e,k1,alpha)

b=k1;

ABS = abs(e);
SGN = e ./ (ABS + alpha);
u = u1 - b*((ABS.^0.5).*SGN); 

end

== matlab function CAMFC2_04_Quad_03_R2017a/Agent #3/Decenteralized Cooperaive Controller #3/Velocity AMFC #3/Differentiator/Sliding differentiator1 ==
  data: Du1 output; e input; k2 parameter; alpha parameter
function Du1 = fcn(e,k2,alpha)

a=k2;

ABS = abs(e);
SGN = e ./ (ABS + alpha);
Du1 = - a*SGN;

end

== matlab function CAMFC2_04_Quad_03_R2017a/Agent #3/Decenteralized Cooperaive Controller #3/Velocity AMFC #3/g-Estimator ==
  data: sigma input; g_hat input; P input; rho_1v parameter; gamma_1v parameter; Dg_hat output
function Dg_hat = fcn(sigma,g_hat,P,rho_1v,gamma_1v)

Dg_hat = - gamma_1v * P * sigma - rho_1v * gamma_1v * g_hat;

end

== matlab function CAMFC2_04_Quad_03_R2017a/Agent #3/Decenteralized Cooperaive Controller #3/Velocity AMFC #3/main ==
  data: sigma input; zeta input; u output; Dy_d input; Rv parameter; P input; a_hat input; Bv parameter; g_hat input; x input; Qv parameter; BvBT_inv parameter; n0 parameter
function u = fcn(sigma,zeta,Dy_d,Rv,P,a_hat,Bv,g_hat,x,Qv,BvBT_inv,n0)

u1 = (1/2) * Rv * Bv' * P * sigma;
u2 = BvBT_inv * (Dy_d - a_hat*x + (eye(n0) + 2*(((P)^(-1)*Qv)) + a_hat)*sigma - g_hat - zeta) - (3/4) * Rv * Bv' * P * sigma;

u = u1 + u2;

end

== matlab function CAMFC2_04_Quad_03_R2017a/Agent #3/Decenteralized Cooperaive Controller #3/Velocity AMFC #3/variable change ==
  data: X input; Xd input; x_mod output; xd_mod output; e_mod output
function [x_mod,xd_mod,e_mod] = fcn(X,Xd)

x_mod = X;
xd_mod = Xd;
e_mod = xd_mod - x_mod;

end

== matlab function CAMFC2_04_Quad_03_R2017a/Agent #3/Plant #3/MATLAB Function ==
  data: XT_V input; XR input; U input; t input; DP output; Dv output; Kd parameter; Ka parameter; M parameter; J parameter; ge parameter; DXR output; noise_amp parameter; noise_frq parameter
function [DP,Dv,DXR] = fcn(XT_V,XR,U,t,Kd,Ka,M,J,ge,noise_amp, noise_frq)

phi = XR(1);
theta = XR(2);
psi = XR(3);

Rq = [cos(psi)*cos(theta) -sin(psi)*cos(phi)+cos(psi)*sin(theta)*sin(phi) sin(psi)*sin(phi)+cos(psi)*sin(theta)*cos(phi);
    sin(psi)*cos(theta) cos(psi)*cos(phi)+sin(psi)*sin(theta)*sin(phi) -cos(psi)*sin(phi)+sin(psi)*sin(theta)*cos(phi);
    -sin(theta) cos(theta)*sin(phi) cos(theta)*cos(phi)]; 

R_omega = [1 0 -sin(theta);
    0 cos(phi) cos(theta)*sin(phi);
    0 -sin(phi) cos(theta)*cos(phi)];

EXT_PRD = External_Product3(XR(4:6),(J*XR(4:6)));

FTT = Rq * [0;0;U(1)];
TTT = U(2:4);

DP = XT_V;
DPHI = (R_omega)^(-1) * XR(4:6); 
Dv = (1/M)*(FTT - Kd*XT_V - M*[0;0;ge] + Rq*(noise_amp*sin(noise_frq*t))*[0;0;1]); 
Dw = (J^(-1))*(TTT - Ka*XR(4:6) - EXT_PRD + (noise_amp*sin(noise_frq*t)*[1;1;1]));
DXR = [DPHI;Dw];

end

== matlab function CAMFC2_04_Quad_03_R2017a/Agent #4/Decenteralized Cooperaive Controller #4/Controller to Motors #4 ==
  data: u output; uT input; uR input
function u = fcn(uT,uR)

y1 = uR(4);
y2 = uR(5);
y3 = uR(6);

Y = [uT;y1;y2;y3];

u = Y;

end
